simulink subsystem "stack_subsystem_model"  (R2023a)
settings: Solver=VariableStepAuto  StartTime=0.0  StopTime=10.0  RelTol=1e-3
values from neighbouring files (symbols this model uses):
  constants =     [All_Properties.mat]
  coolant_initial_temperature = 313.15    [All_Properties.mat]    (also in cathode_subsystem_parameters.m = 293.15; thermal_subsystem_parameters.m = 293.15)
  coolant_num_layers = 20    [All_Properties.mat]    (also in Plant_Model_HT_Cooling_Parameters.m; cathode_subsystem_parameters.m = 15; environment_parameters.m; stack_model_harness_parameters.m)
  coolant_num_passes = 12    [All_Properties.mat]    (also in Plant_Model_HT_Cooling_Parameters.m; cathode_subsystem_parameters.m = 20; environment_parameters.m; stack_model_harness_parameters.m)
  coolant_w_channels = 1    [All_Properties.mat]    (also in Plant_Model_HT_Cooling_Parameters.m; cathode_subsystem_parameters.m; environment_parameters.m; stack_model_harness_parameters.m)
  env_p = 0.101325    [All_Properties.mat]    (also in Plant_Model_HT_Cooling_Parameters.m; anode_subsystem_parameters.m; environment_parameters.m; stack_model_harness_parameters.m)
  hydrogen =     [All_Properties.mat]
  oxygen =     [All_Properties.mat]
  stack_area = 300    [All_Properties.mat]    (also in Plant_Model_HT_Cooling_Parameters.m = 280; cathode_subsystem_parameters.m = 280; stack_model_parameters.m = 280; stack_subsystem_parameters.m)
  stack_num_cells = 455    [All_Properties.mat]    (also in Plant_Model_HT_Cooling_Parameters.m = 400; cathode_subsystem_parameters.m; stack_model_parameters.m = 400; stack_subsystem_parameters.m)
undefined symbols (not defined in the file or in its folder): dewpoint_temperature_degC, h2_molar_concentration, inlet_flow_lpmin, inlet_pressure_barg, inlet_temperature_degC, stoichiometry
libraries: fl_lib x39, nesl_utility x31
(part 2 of 2)

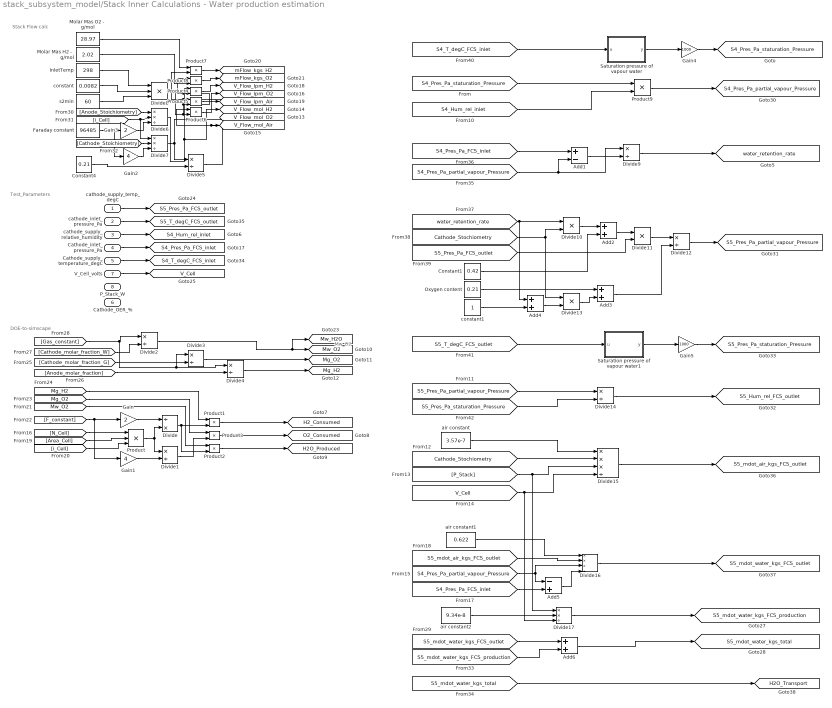
== system stack_subsystem_model/Stack Inner Calculations - Water production estimation ==
  note: Test_Parameters
  note: Mw_O2
  note: Stack Flow calc
  note: DOE-to-simscape
  cathode_supply_temp_degC : Inport
  cathode_inlet_pressure_Pa : Inport  Port=2
  cathode_supply_relative_humidity : Inport  Port=3
  Cathode_inlet_pressure_Pa : Inport  Port=4
  Cathode_supply_temperature_degC : Inport  Port=5
  Cathode_OER_% : Inport  Port=6
  V_Cell_volts : Inport  Port=7
  P_Stack_W : Inport  Port=8
  Add1 : Sum  Inputs=+-
  Add{2..4,6} (4 alike) : Sum
  Add5 : Sum  Inputs=-+
  Constant1 : Constant  Value=0.42
  Constant4 : Constant  Value=0.21
  Divide : Product  Inputs=/*
  Divide{1..5,9,12,14} (8 alike) : Product  Inputs=*/
  Divide10 : Product  Inputs=**
  Divide11 : Product  Inputs=**
  Divide13 : Product  Inputs=**
  Divide15 : Product  Inputs=***/
  Divide16 : Product  Inputs=***/
  Divide17 : Product  Inputs=**/
  Divide6 : Product  Inputs=**/
  Divide7 : Product  Inputs=**/
  Divide8 : Product  Inputs=***
  Faraday constant : Constant  Value=96485
  Gain : Gain  Gain=2
  Gain1 : Gain  Gain=4
  Gain2 : Gain  Gain=4
  Gain3 : Gain  Gain=2
  Gain4 : Gain  Gain=1000
  Gain5 : Gain  Gain=1000
  InletTemp : Constant  Value=298
  Molar Mas H2 -  g/mol : Constant  Value=2.02
  "Molar Mas O2 -  g/mol " : Constant  Value=28.97
  Oxygen content : Constant  Value=0.21
  Product : Product  Inputs=3
  Product{1..9} (9 alike) : Product
  Saturation pressure of vapour water : MATLAB Function  TreatAsAtomicUnit=on
  Saturation pressure of vapour water1 : MATLAB Function  TreatAsAtomicUnit=on
  air constant : Constant  Value=3.57e-7
  air constant1 : Constant  Value=0.622
  air constant2 : Constant  Value=9.34e-8
  constant : Constant  Value=0.0082
  constant1 : Constant
  s2min : Constant  Value=60
  tag scope: H2O_Produced=global, H2O_Transport=global, H2_Consumed=global, Mg_H2=global, Mg_O2=global, Mw_H2O=global, Mw_O2=global, O2_Consumed=global, S4_Hum_rel_inlet=global, S4_Pres_Pa_FCS_inlet=global, S4_Pres_Pa_partial_vapour_Pressure=global, S4_Pres_Pa_staturation_Pressure=global, S4_T_degC_FCS_inlet=global, S5_Hum_rel_FCS_outlet=global, S5_Pres_Pa_FCS_outlet=global, S5_Pres_Pa_partial_vapour_Pressure=global, S5_Pres_Pa_staturation_Pressure=global, S5_T_degC_FCS_outlet=global, S5_mdot_air_kgs_FCS_outlet=global, S5_mdot_water_kgs_FCS_outlet=global, S5_mdot_water_kgs_FCS_production=global, S5_mdot_water_kgs_total=global, V_Cell=global, V_Flow_lpm_Air=global, V_Flow_lpm_H2=global, V_Flow_lpm_O2=global, V_Flow_mol_Air=global, V_Flow_mol_H2=global, V_Flow_mol_O2=global, mFlow_kgs_H2=global, mFlow_kgs_O2=global, water_retention_rate=global
  wires:
  [S5_Pres_Pa_staturation_Pressure] -> Divide14/2
  cathode_supply_relative_humidity/1 -> [S4_Hum_rel_inlet]
  [V_Cell] -> Divide15/4, Divide17/3
  Divide10/1 -> Add2/1
  Divide14/1 -> [S5_Hum_rel_FCS_outlet]
  Divide17/1 -> [S5_mdot_water_kgs_FCS_production]
  Divide12/1 -> [S5_Pres_Pa_partial_vapour_Pressure]
  air constant1/1 -> Divide16/1
  Divide16/1 -> [S5_mdot_water_kgs_FCS_outlet]
  [S4_Pres_Pa_FCS_inlet] -> Add1/1
  Cathode_inlet_pressure_Pa/1 -> [S4_Pres_Pa_FCS_inlet]
  Add3/1 -> Divide12/2
  [S4_Pres_Pa_FCS_inlet] -> Add5/2
  V_Cell_volts/1 -> [V_Cell]
  [S4_T_degC_FCS_inlet] -> Saturation pressure of vapour water/1(u)
  Add1/1 -> Divide9/2
  Divide9/1 -> [water_retention_rate]
  Divide15/1 -> [S5_mdot_air_kgs_FCS_outlet]
  Oxygen content/1 -> Add3/1
  Add4/1 -> Divide13/2
  Cathode_supply_temperature_degC/1 -> [S4_T_degC_FCS_inlet]
  Saturation pressure of vapour water/1(y) -> Gain4/1
  Add6/1 -> [S5_mdot_water_kgs_total]
  [S5_Pres_Pa_FCS_outlet] -> Divide11/2
  cathode_supply_temp_degC/1 -> [S5_Pres_Pa_FCS_outlet]
  constant1/1 -> Add4/2
  [S5_mdot_water_kgs_FCS_production] -> Add6/2
  Divide11/1 -> Divide12/1
  Add5/1 -> Divide16/4
  [S4_Pres_Pa_staturation_Pressure] -> Product9/1
  [S4_Hum_rel_inlet] -> Product9/2
  cathode_inlet_pressure_Pa/1 -> [S5_T_degC_FCS_outlet]
  air constant2/1 -> Divide17/2
  [P_Stack] -> Divide15/3, Divide17/1
  [S5_mdot_water_kgs_total] -> [H2O_Transport]
  Divide13/1 -> Add3/2
  [S5_Pres_Pa_partial_vapour_Pressure] -> Divide14/1
  [S5_T_degC_FCS_outlet] -> Saturation pressure of vapour water1/1(u)
  [Cathode_Stochiometry] -> Divide15/2
  [S5_mdot_water_kgs_FCS_outlet] -> Add6/1
  Saturation pressure of vapour water1/1(y) -> Gain5/1
  [S4_Pres_Pa_partial_vapour_Pressure] -> Add1/2, Divide9/1
  Constant1/1 -> Add2/2
  Add2/1 -> Divide11/1
  Gain4/1 -> [S4_Pres_Pa_staturation_Pressure]
  [water_retention_rate] -> Add4/1, Divide10/1
  [Cathode_Stochiometry] -> Divide10/2, Divide13/1
  [S4_Pres_Pa_partial_vapour_Pressure] -> Add5/1, Divide16/3
  Product9/1 -> [S4_Pres_Pa_partial_vapour_Pressure]
  air constant/1 -> Divide15/1
  Gain5/1 -> [S5_Pres_Pa_staturation_Pressure]
  [S5_mdot_air_kgs_FCS_outlet] -> Divide16/2
  [Cathode_molar_fraction_W] -> Divide2/2
  Product/1 -> Divide/2, Divide1/1
  [Area_Cell] -> Product/2
  Divide6/1 -> [V_Flow_mol_H2], Product4/1
  Product8/1 -> [mFlow_kgs_O2]
  [Gas_constant] -> Divide3/1, Divide4/1, Divide2/1
  [N_Cell] -> Product/1
  constant/1 -> Divide8/2
  [Cathode_Stoichiometry] -> Divide7/2
  Divide8/1 -> Product8/1, Product4/2, Product5/2, Product6/2
  Product1/1 -> [H2_Consumed]
  Divide7/1 -> [V_Flow_mol_O2], Product7/2, Product5/1, Divide5/1
  Gain3/1 -> Divide6/3
  Faraday constant/1 -> Gain3/1, Gain2/1
  [i_Cell] -> Divide6/2, Divide7/1
  Gain/1 -> Divide/1
  [i_Cell] -> Product/3
  Gain1/1 -> Divide1/2
  [F_constant] -> Gain1/1, Gain/1
  [Anode_molar_fraction] -> Divide4/2
  [Cathode_molar_fraction_G] -> Divide3/2
  Divide2/1 -> [Mw_H2O], [Mw_O2]
  Divide5/1 -> Product6/1, [V_Flow_mol_Air]
  Divide3/1 -> [Mg_O2]
  Divide4/1 -> [Mg_H2]
  Gain2/1 -> Divide7/3
  Constant4/1 -> Divide5/2
  [Anode_Stoichiometry] -> Divide6/1
  InletTemp/1 -> Divide8/1
  s2min/1 -> Divide8/3
  Product4/1 -> [V_Flow_lpm_H2]
  Product5/1 -> [V_Flow_lpm_O2]
  Product7/1 -> [mFlow_kgs_H2]
  Molar Mas H2 -  g/mol/1 -> Product8/2
  Product2/1 -> [H2O_Produced]
  "Molar Mas O2 -  g/mol "/1 -> Product7/1
  Product6/1 -> [V_Flow_lpm_Air]
  Product3/1 -> [O2_Consumed]
  [Mg_H2] -> Product1/1
  [Mw_O2] -> Product2/1
  [Mg_O2] -> Product3/1
  Divide/1 -> Product2/2, Product1/2
  Divide1/1 -> Product3/2

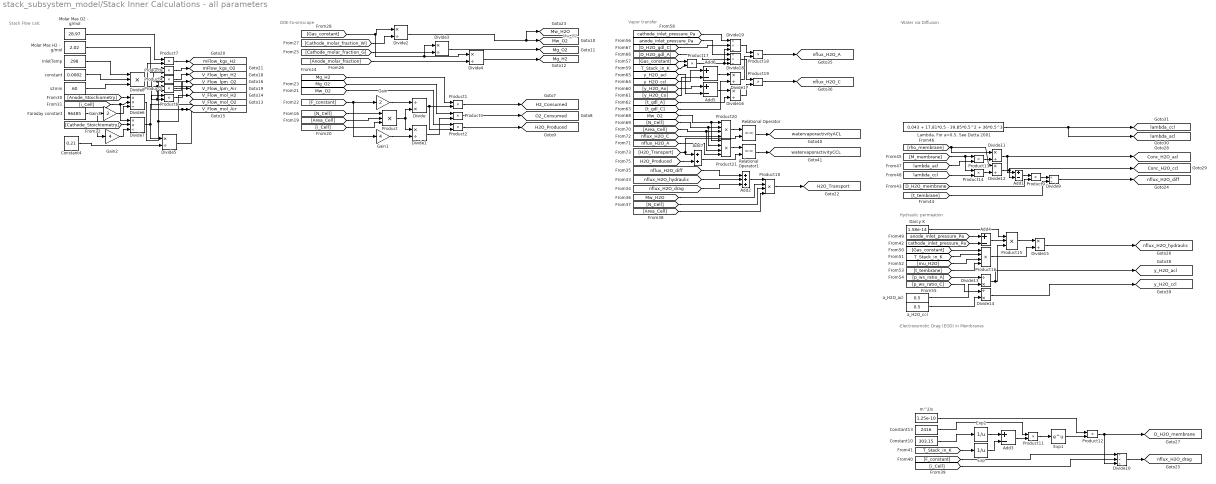
== system stack_subsystem_model/Stack Inner Calculations - all parameters ==
  note: Hydraulic permeation
  note: -Electroosmotic Drag (EOD) in Membranes
  note: DOE-to-simscape
  note: Stack Flow calc
  note: Mw_O2
  note: -Water via Diffusion
  note: Vapor transfer
  Add{1,3..6} (5 alike) : Sum  Inputs=+-
  Add2 : Sum  Inputs=+++
  Add7 : Sum
  Constant10 : Constant  Value=303.15
  Constant13 : Constant  Value=2416
  Constant4 : Constant  Value=0.21
  Darcy K : Constant  Value=1.58e-14
  Divide : Product  Inputs=/*
  Divide{1..5,9,11..12,15..17} (11 alike) : Product  Inputs=*/
  Divide10 : Product  Inputs=/**
  Divide13 : Product  Inputs=/*
  Divide14 : Product  Inputs=/*
  Divide{6..7,18..19} (4 alike) : Product  Inputs=**/
  Divide8 : Product  Inputs=***
  Exp : Math  Operator=reciprocal
  Exp1 : Math
  Exp2 : Math  Operator=reciprocal
  Faraday constant : Constant  Value=96485
  Gain : Gain  Gain=2
  Gain1 : Gain  Gain=4
  Gain2 : Gain  Gain=4
  Gain3 : Gain  Gain=2
  InletTemp : Constant  Value=298
  "Lambda, For a=0.5, See Dutta 2001" : Constant  Value=0.043 + 17.81*0.5 - 39.85*0.5^2 + 36*0.5^3
  Molar Mas H2 -  g/mol : Constant  Value=2.02
  "Molar Mas O2 -  g/mol " : Constant  Value=28.97
  Product : Product  Inputs=3
  Product{1..9,11..14,17..19} (16 alike) : Product
  Product{10,16,20..21} (4 alike) : Product  Inputs=4
  Product15 : Product  Inputs=3
  Relational Operator : RelationalOperator  Operator===  OutDataTypeStr=boolean  RndMeth=Simplest  InputSameDT=off
  Relational Operator1 : RelationalOperator  Operator===  OutDataTypeStr=boolean  RndMeth=Simplest  InputSameDT=off
  a_H2O_acl : Constant  Value=0.5
  a_H2O_ccl : Constant  Value=0.5
  constant : Constant  Value=0.0082
  m^2/s : Constant  Value=1.25e-10
  s2min : Constant  Value=60
  tag scope: Conc_H2O_acl=global, Conc_H2O_ccl=global, D_H2O_membrane=global, H2O_Produced=global, H2O_Transport=global, H2_Consumed=global, Mg_H2=global, Mg_O2=global, Mw_H2O=global, Mw_O2=global, O2_Consumed=global, V_Flow_lpm_Air=global, V_Flow_lpm_H2=global, V_Flow_lpm_O2=global, V_Flow_mol_Air=global, V_Flow_mol_H2=global, V_Flow_mol_O2=global, lambda_acl=global, lambda_ccl=global, mFlow_kgs_H2=global, mFlow_kgs_O2=global, nflux_H2O_A=global, nflux_H2O_C=global, nflux_H2O_diff=global, nflux_H2O_drag=global, nflux_H2O_hydraulic=global, watervaporactivityACL=global, watervaporactivityCCL=global, y_H2O_acl=global, y_H2O_ccl=global
  wires:
  a_H2O_acl/1 -> Divide13/2
  Darcy K/1 -> Product15/1
  Add4/1 -> Product15/2
  [cathode_inlet_pressure_Pa] -> Add4/2
  [anode_inlet_pressure_Pa] -> Add4/1
  Product14/1 -> Divide12/2
  Divide15/1 -> [nflux_H2O_hydraulic]
  Product16/1 -> Divide15/2
  [lambda_ccl] -> Product14/2
  Product15/1 -> Divide15/1
  [mu_H2O] -> Product16/3
  [t_tembrane] -> Product16/4
  a_H2O_ccl/1 -> Divide14/2
  [p_ws_ratio_A] -> Divide13/1
  [p_ws_ratio_C] -> Divide14/1
  Divide1/1 -> Product3/2
  Divide/1 -> Product1/2, Product2/2
  [Mg_O2] -> Product3/1
  [Mw_O2] -> Product2/1
  [Mg_H2] -> Product1/1
  Product3/1 -> [O2_Consumed]
  Product6/1 -> [V_Flow_lpm_Air]
  "Molar Mas O2 -  g/mol "/1 -> Product7/1
  Product2/1 -> [H2O_Produced]
  Molar Mas H2 -  g/mol/1 -> Product8/2
  Product7/1 -> [mFlow_kgs_H2]
  Product5/1 -> [V_Flow_lpm_O2]
  Product4/1 -> [V_Flow_lpm_H2]
  s2min/1 -> Divide8/3
  InletTemp/1 -> Divide8/1
  [Anode_Stoichiometry] -> Divide6/1
  Constant4/1 -> Divide5/2
  Gain2/1 -> Divide7/3
  Divide4/1 -> [Mg_H2]
  Divide3/1 -> [Mg_O2]
  Divide5/1 -> [V_Flow_mol_Air], Product6/1
  Divide2/1 -> [Mw_O2], [Mw_H2O]
  [Cathode_molar_fraction_G] -> Divide3/2
  [Anode_molar_fraction] -> Divide4/2
  [F_constant] -> Gain/1, Gain1/1
  Gain1/1 -> Divide1/2
  [i_Cell] -> Product/3
  Gain/1 -> Divide/1
  [y_H2O_Ao] -> Add5/1
  [i_Cell] -> Divide7/1, Divide6/2
  Faraday constant/1 -> Gain2/1, Gain3/1
  Gain3/1 -> Divide6/3
  Divide7/1 -> Divide5/1, Product5/1, Product7/2, [V_Flow_mol_O2]
  Relational Operator/1 -> [watervaporactivityACL]
  "Lambda, For a=0.5, See Dutta 2001"/1 -> [lambda_ccl], [lambda_acl]
  Relational Operator1/1 -> [watervaporactivityCCL]
  [H2O_Produced] -> Add7/2
  [nflux_H2O_A] -> Product21/4
  Product21/1 -> Relational Operator1/1
  Product20/1 -> Relational Operator/1
  [nflux_H2O_C] -> Product20/4
  [H20_Transport] -> Add7/1, Relational Operator/2
  [Area_Cell] -> Product20/3, Product21/3
  [cathode_inlet_pressure_Pa] -> Divide19/1
  Divide18/1 -> Product19/1
  Divide17/1 -> Product18/2
  [T_Stack_in_K] -> Product17/2
  Product18/1 -> [nflux_H2O_A]
  [t_gdl_C] -> Divide17/2
  [nflux_H2O_hydraulic] -> Add2/2
  Divide19/1 -> Product18/1
  Product1/1 -> [H2_Consumed]
  [Mw_O2] -> Product20/1, Product21/1
  [Gas_constant] -> Product16/1
  Product19/1 -> [nflux_H2O_C]
  Add6/1 -> Divide17/1
  [t_tembrane] -> Divide9/2
  [anode_inlet_pressure_Pa] -> Divide18/1
  Divide8/1 -> Product6/2, Product5/2, Product4/2, Product8/1
  Product10/1 -> [H2O_Transport]
  [Gas_constant] -> Product17/1
  [Cathode_Stoichiometry] -> Divide7/2
  constant/1 -> Divide8/2
  Divide13/1 -> Product15/3, [y_H2O_acl]
  [y_H2O_ccl] -> Add6/1
  Add2/1 -> Product10/1
  [D_H2O_gdl_C] -> Divide19/2
  [N_Cell] -> Product/1
  [M_membrane] -> Product14/1, Product13/1
  [D_H2O_gdl_A] -> Divide18/2
  [lambda_acl] -> Product13/2
  [Gas_constant] -> Divide2/1, Divide4/1, Divide3/1
  Divide9/1 -> [nflux_H2O_diff]
  Divide16/1 -> Product19/2
  [N_Cell] -> Product20/2, Product21/2
  Product8/1 -> [mFlow_kgs_O2]
  Add5/1 -> Divide16/1
  Constant13/1 -> Product11/1
  Divide6/1 -> Product4/1, [V_Flow_mol_H2]
  Product11/1 -> Exp1/1
  m^2/s/1 -> Product12/1
  Exp2/1 -> Add3/1
  [Mw_H2O] -> Product10/2
  Product17/1 -> Divide18/3, Divide19/3
  Divide10/1 -> [nflux_H2O_drag]
  Exp/1 -> Add3/2
  Product13/1 -> Divide11/2
  [T_Stack_in_K] -> Exp/1
  Add3/1 -> Product11/2
  [Area_Cell] -> Product/2
  [D_H2O_membrane] -> Product9/2
  [t_gdl_A] -> Divide16/2
  [T_Stack_in_K] -> Product16/2
  Exp1/1 -> Product12/2
  [i_Cell] -> Divide10/2
  Divide11/1 -> Add1/1, [Conc_H2O_acl]
  [Area_Cell] -> Product10/4
  [y_H2O_acl] -> Add5/2
  [y_H2O_Co] -> Add6/2
  Constant10/1 -> Exp2/1
  Product/1 -> Divide1/1, Divide/2
  [nflux_H2O_drag] -> Add2/3
  Product12/1 -> [D_H2O_membrane], Divide10/3
  Add7/1 -> Relational Operator1/2
  Add1/1 -> Product9/1
  [nflux_H2O_diff] -> Add2/1
  [N_Cell] -> Product10/3
  [Cathode_molar_fraction_W] -> Divide2/2
  Divide12/1 -> [Conc_H2O_ccl], Add1/2
  Divide14/1 -> [y_H2O_ccl]
  [F_constant] -> Divide10/1
  [rho_membrane] -> Divide11/1, Divide12/1
  Product9/1 -> Divide9/1

== matlab function stack_subsystem_model/Simulink Function/MATLAB Function ==
  data: moist_air_temperature input; relative_humidity input; dewpoint_temperature output
function dewpoint_temperature = approximate_dewpoint(moist_air_temperature, relative_humidity)
% This function approximates the dewpoint temperature of moist air
% according to the August–Roche–Magnus approximation of the
% Clausius–Clapeyron equation.
%
% Inputs: Relative Humidity [-], Moist Air Temperature [°C]
% Output: Dewpoint Temperature [°C]
%
% Reference: https://bmcnoldy.earth.miami.edu/Humidity.html, retrieved
% 09/07/2023

% clip to [0, 1] and convert to [%]
relative_humidity = min(max(0, relative_humidity), 1)*100;

% August–Roche–Magnus approximation
dewpoint_temperature = 243.04*(log(relative_humidity/100)+((17.625*moist_air_temperature)/(243.04+moist_air_temperature)))/...
    (17.625-log(relative_humidity/100)-((17.625*moist_air_temperature)/(243.04+moist_air_temperature)));

== matlab function stack_subsystem_model/evaluate_doe_model ==
  data: current input; anode_pressure_drop_mbar output; anode_temp_delta_degC output; cathode_pressure_drop_mbar output; cathode_temp_delta_degC output; cell_voltage_max_V output; cell_voltage_mean_V output; cell_voltage_min_V output; cell_voltage_std_dev_mV output; coolant_pressure_drop_mbar output; coolant_temp_delta_degC output; stack_voltage_V output; anode_supply input; stack_voltage_loss_V output; cathode_supply input; coolant_supply input
function [anode_pressure_drop_mbar, anode_temp_delta_degC, cathode_pressure_drop_mbar, ...
cathode_temp_delta_degC, cell_voltage_max_V, cell_voltage_mean_V, cell_voltage_min_V, ...
cell_voltage_std_dev_mV, coolant_pressure_drop_mbar, coolant_temp_delta_degC, ...
stack_voltage_V, stack_voltage_loss_V] = evaluate_doe_model(current, anode_supply, cathode_supply, coolant_supply)

% This function calls the .mex files created from PowerCell response
% surface interpolation of DoE data by providing the input arguments: 
% [current, anode_supply, cathode_supply, coolant_supply]. Note that the
% "model is only valid within the range of tested data." For more
% information, see: p10_doe_files\vendor_provision\Stack_Data_Model_Information.pdf

%% exclude .mex files from code generation

coder.extrinsic('get_anode_pressure_drop', 'get_anode_temp_delta', ...
    'get_cathode_pressure_drop', 'get_cathode_temp_delta', 'get_cell_voltage_max', ...
    'get_cell_voltage_mean', 'get_cell_voltage_min', 'get_cell_voltage_std_dev', ...
    'get_coolant_pressure_drop', 'get_coolant_temp_delta', 'get_stack_voltage', ...
    'get_stack_voltage_loss')

%% instantiate .mex file return variables as doubles

anode_pressure_drop_mbar = double(0);
anode_temp_delta_degC = double(0);
cathode_pressure_drop_mbar = double(0);
cathode_temp_delta_degC = double(0);
cell_voltage_max_V = double(0);
cell_voltage_mean_V = double(0);
cell_voltage_min_V = double(0);
cell_voltage_std_dev_mV = double(0);
coolant_pressure_drop_mbar = double(0);
coolant_temp_delta_degC = double(0);
stack_voltage_V = double(0);
stack_voltage_loss_V = double(0);

%% call .mex files created from PowerCell response surface interpolation of DoE data

anode_pressure_drop_mbar = get_anode_pressure_drop(current, ...
    anode_supply.h2_molar_concentration, anode_supply.stoichiometry, anode_supply.dewpoint_temperature_degC, anode_supply.inlet_temperature_degC, anode_supply.inlet_pressure_barg, ...
    cathode_supply.stoichiometry, cathode_supply.dewpoint_temperature_degC, cathode_supply.inlet_temperature_degC, cathode_supply.inlet_pressure_barg, ...
    coolant_supply.inlet_flow_lpmin, coolant_supply.inlet_temperature_degC);
anode_temp_delta_degC = get_anode_temp_delta(current, ...
    anode_supply.h2_molar_concentration, anode_supply.stoichiometry, anode_supply.dewpoint_temperature_degC, anode_supply.inlet_temperature_degC, anode_supply.inlet_pressure_barg, ...
    cathode_supply.stoichiometry, cathode_supply.dewpoint_temperature_degC, cathode_supply.inlet_temperature_degC, cathode_supply.inlet_pressure_barg, ...
    coolant_supply.inlet_flow_lpmin, coolant_supply.inlet_temperature_degC);
cathode_pressure_drop_mbar = get_cathode_pressure_drop(current, ...
    anode_supply.h2_molar_concentration, anode_supply.stoichiometry, anode_supply.dewpoint_temperature_degC, anode_supply.inlet_temperature_degC, anode_supply.inlet_pressure_barg, ...
    cathode_supply.stoichiometry, cathode_supply.dewpoint_temperature_degC, cathode_supply.inlet_temperature_degC, cathode_supply.inlet_pressure_barg, ...
    coolant_supply.inlet_flow_lpmin, coolant_supply.inlet_temperature_degC);
cathode_temp_delta_degC = get_cathode_temp_delta(current, ...
    anode_supply.h2_molar_concentration, anode_supply.stoichiometry, anode_supply.dewpoint_temperature_degC, anode_supply.inlet_temperature_degC, anode_supply.inlet_pressure_barg, ...
    cathode_supply.stoichiometry, cathode_supply.dewpoint_temperature_degC, cathode_supply.inlet_temperature_degC, cathode_supply.inlet_pressure_barg, ...
    coolant_supply.inlet_flow_lpmin, coolant_supply.inlet_temperature_degC);
cell_voltage_max_V = get_cell_voltage_max(current, ...
    anode_supply.h2_molar_concentration, anode_supply.stoichiometry, anode_supply.dewpoint_temperature_degC, anode_supply.inlet_temperature_degC, anode_supply.inlet_pressure_barg, ...
    cathode_supply.stoichiometry, cathode_supply.dewpoint_temperature_degC, cathode_supply.inlet_temperature_degC, cathode_supply.inlet_pressure_barg, ...
    coolant_supply.inlet_flow_lpmin, coolant_supply.inlet_temperature_degC);
cell_voltage_mean_V = get_cell_voltage_mean(current, ...
    anode_supply.h2_molar_concentration, anode_supply.stoichiometry, anode_supply.dewpoint_temperature_degC, anode_supply.inlet_temperature_degC, anode_supply.inlet_pressure_barg, ...
    cathode_supply.stoichiometry, cathode_supply.dewpoint_temperature_degC, cathode_supply.inlet_temperature_degC, cathode_supply.inlet_pressure_barg, ...
    coolant_supply.inlet_flow_lpmin, coolant_supply.inlet_temperature_degC);
cell_voltage_min_V = get_cell_voltage_min(current, ...
    anode_supply.h2_molar_concentration, anode_supply.stoichiometry, anode_supply.dewpoint_temperature_degC, anode_supply.inlet_temperature_degC, anode_supply.inlet_pressure_barg, ...
    cathode_supply.stoichiometry, cathode_supply.dewpoint_temperature_degC, cathode_supply.inlet_temperature_degC, cathode_supply.inlet_pressure_barg, ...
    coolant_supply.inlet_flow_lpmin, coolant_supply.inlet_temperature_degC);
cell_voltage_std_dev_mV = get_cell_voltage_std_dev(current, ...
    anode_supply.h2_molar_concentration, anode_supply.stoichiometry, anode_supply.dewpoint_temperature_degC, anode_supply.inlet_temperature_degC, anode_supply.inlet_pressure_barg, ...
    cathode_supply.stoichiometry, cathode_supply.dewpoint_temperature_degC, cathode_supply.inlet_temperature_degC, cathode_supply.inlet_pressure_barg, ...
    coolant_supply.inlet_flow_lpmin, coolant_supply.inlet_temperature_degC);
coolant_pressure_drop_mbar = get_coolant_pressure_drop(current, ...
    anode_supply.h2_molar_concentration, anode_supply.stoichiometry, anode_supply.dewpoint_temperature_degC, anode_supply.inlet_temperature_degC, anode_supply.inlet_pressure_barg, ...
    cathode_supply.stoichiometry, cathode_supply.dewpoint_temperature_degC, cathode_supply.inlet_temperature_degC, cathode_supply.inlet_pressure_barg, ...
    coolant_supply.inlet_flow_lpmin, coolant_supply.inlet_temperature_degC);
coolant_temp_delta_degC = get_coolant_temp_delta(current, ...
    anode_supply.h2_molar_concentration, anode_supply.stoichiometry, anode_supply.dewpoint_temperature_degC, anode_supply.inlet_temperature_degC, anode_supply.inlet_pressure_barg, ...
    cathode_supply.stoichiometry, cathode_supply.dewpoint_temperature_degC, cathode_supply.inlet_temperature_degC, cathode_supply.inlet_pressure_barg, ...
    coolant_supply.inlet_flow_lpmin, coolant_supply.inlet_temperature_degC);
stack_voltage_V = get_stack_voltage(current, ...
    anode_supply.h2_molar_concentration, anode_supply.stoichiometry, anode_supply.dewpoint_temperature_degC, anode_supply.inlet_temperature_degC, anode_supply.inlet_pressure_barg, ...
    cathode_supply.stoichiometry, cathode_supply.dewpoint_temperature_degC, cathode_supply.inlet_temperature_degC, cathode_supply.inlet_pressure_barg, ...
    coolant_supply.inlet_flow_lpmin, coolant_supply.inlet_temperature_degC);
stack_voltage_loss_V = get_stack_voltage_loss(current, ...
    anode_supply.h2_molar_concentration, anode_supply.stoichiometry, anode_supply.dewpoint_temperature_degC, anode_supply.inlet_temperature_degC, anode_supply.inlet_pressure_barg, ...
    cathode_supply.stoichiometry, cathode_supply.dewpoint_temperature_degC, cathode_supply.inlet_temperature_degC, cathode_supply.inlet_pressure_barg, ...
    coolant_supply.inlet_flow_lpmin, coolant_supply.inlet_temperature_degC);

== matlab function stack_subsystem_model/Stack Inner Calculations - Water production estimation/Saturation pressure of vapour water ==
  data: u input; y output
function y = fcn(u)

y =  0.61121 * exp((18.678 - (u / 234.5)) * (u / (257.14 + u)));;

== matlab function stack_subsystem_model/Stack Inner Calculations - Water production estimation/Saturation pressure of vapour water1 ==
  data: u input; y output
function y = fcn(u)

y =  0.61121 * exp((18.678 - (u / 234.5)) * (u / (257.14 + u)));;
